simulink model "Simulink_DB2"  (R2012b)
settings: Solver=ode3  StartTime=0.0  StopTime=inf  FixedStep=0.001  RelTol=1e-3
undefined symbols (not defined in the file or in its folder): NULL
libraries: instrumentlib x3
settings Model: Creator=Petito  LastModifiedBy=Augusto
settings DataIOCC: SignalLoggingSaveFormat=ModelDataLogs
settings OptimizationCC: ExpressionDepthLimit=128
settings DebuggingCC: MultiTaskDSMMsg=warning  MultiTaskCondExecSysMsg=none  StrictBusMsg=None
settings HardwareCC: ProdIntDivRoundTo=Zero  ProdEndianess=LittleEndian  ProdHWDeviceType=Generic->32-bit x86 compatible
settings RTWCC: SystemTargetFile=rtwin.tlc  TemplateMakefile=rtwin.tmf  Description=Real-Time Windows Target  ProcessScript=rtwin_make_rtw_hook  IncludeERTFirstTime=on  RTWCompilerOptimization=On
settings CodeAppCC: MaxIdLength=95  CustomSymbolStrType=$N$R$M_T  InternalIdentifier=Shortened
settings TargetCC: TargetLibSuffix=_rtwin.lib  TargetPreCompLibLocation=C:\Program Files\MATLAB\R2013a\toolbox\rtw\targets\rtwin\lib\win64  CodeReplacementLibrary=ANSI_C  IsPILTarget=off  EnableShiftOperators=on

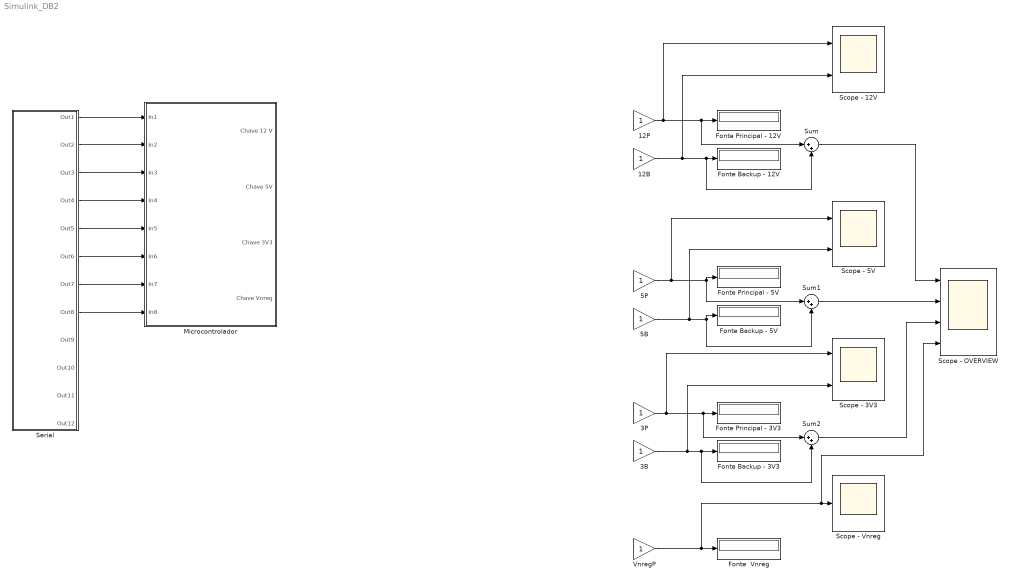
== system Simulink_DB2 ==
  12B : Gain
  12P : Gain
  3B : Gain
  3P : Gain
  5B : Gain
  5P : Gain
  Fonte  Vnreg : Display  mask(a){}
  Fonte Backup - 12V : Display
  Fonte Backup - 3V3 : Display
  Fonte Backup - 5V : Display
  Fonte Principal - 12V : Display  mask(a){}
  Fonte Principal - 3V3 : Display  mask(a){}
  Fonte Principal - 5V : Display  mask(a){}
  Microcontrolador : Subsystem
  Scope - 12V : Scope  NumInputPorts=2
      settings: TickLabels=on  TimeRange=10  YMin=0~0  YMax=13~13
  Scope - 3V3 : Scope  NumInputPorts=2
      settings: TickLabels=on  TimeRange=10  YMin=0~0  YMax=13~13  SaveName=ScopeData3
  Scope - 5V : Scope  NumInputPorts=2
      settings: TickLabels=on  TimeRange=10  YMin=0~0  YMax=6~6.5  SaveName=ScopeData2
  Scope - OVERVIEW : Scope  NumInputPorts=4
      settings: TickLabels=on  TimeRange=10  YMin=0~0~0~0  YMax=13~6~4~9
  Scope - Vnreg : Scope
      settings: TickLabels=on  TimeRange=10  YMin=0  YMax=13  SaveName=ScopeData4
  Serial : Subsystem
  Sum : Sum  Inputs=|++
  Sum1 : Sum  Inputs=|++
  Sum2 : Sum  Inputs=|++
  VnregP : Gain
  wires:
  ? -> VnregP/1
  ? -> 3P/1
  ? -> 3B/1
  ? -> 5P/1
  ? -> 5B/1
  ? -> 12B/1
  ? -> 12P/1
  12P/1 -> Scope - 12V/1, Fonte Principal - 12V/1, Sum/1
  12B/1 -> Scope - 12V/2, Sum/2, Fonte Backup - 12V/1
  5P/1 -> Scope - 5V/1, Fonte Principal - 5V/1, Sum1/1
  5B/1 -> Scope - 5V/2, Fonte Backup - 5V/1, Sum1/2
  VnregP/1 -> Scope - OVERVIEW/4, Scope - Vnreg/1, Fonte  Vnreg/1
  Serial/1(Out1) -> Microcontrolador/1(In1)
  Serial/2(Out2) -> Microcontrolador/2(In2)
  Serial/3(Out3) -> Microcontrolador/3(In3)
  Serial/4(Out4) -> Microcontrolador/4(In4)
  Serial/5(Out5) -> Microcontrolador/5(In5)
  Serial/6(Out6) -> Microcontrolador/6(In6)
  Serial/7(Out7) -> Microcontrolador/7(In7)
  Serial/8(Out8) -> Microcontrolador/8(In8)
  Sum/1 -> Scope - OVERVIEW/1
  Sum1/1 -> Scope - OVERVIEW/2
  3P/1 -> Scope - 3V3/1, Sum2/1, Fonte Principal - 3V3/1
  3B/1 -> Scope - 3V3/2, Sum2/2, Fonte Backup - 3V3/1
  Sum2/1 -> Scope - OVERVIEW/3

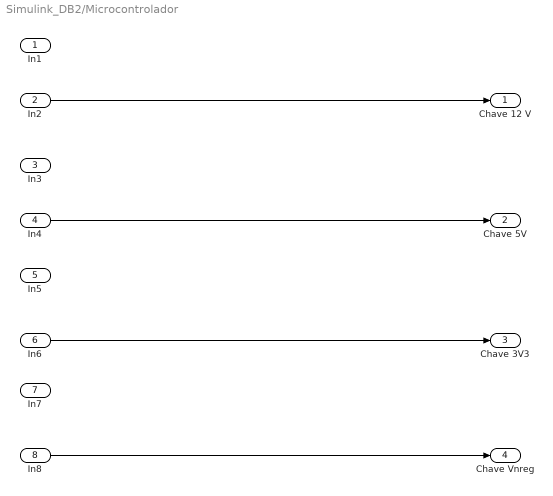
== system Simulink_DB2/Microcontrolador ==
  In1 : Inport
  In2 : Inport  Port=2
  In3 : Inport  Port=3
  In4 : Inport  Port=4
  In5 : Inport  Port=5
  In6 : Inport  Port=6
  In7 : Inport  Port=7
  In8 : Inport  Port=8
  Chave 12 V : Outport
  Chave 5V : Outport  Port=2
  Chave 3V3 : Outport  Port=3
  Chave Vnreg : Outport  Port=4
  wires:
  In4/1 -> Chave 5V/1
  In6/1 -> Chave 3V3/1
  In8/1 -> Chave Vnreg/1
  In2/1 -> Chave 12 V/1

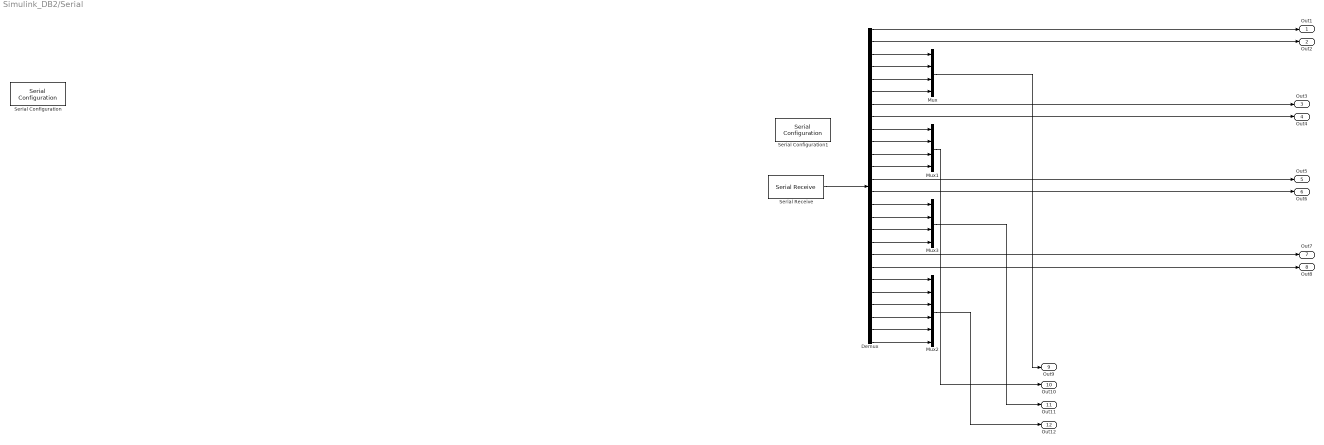
== system Simulink_DB2/Serial ==
  Demux : Demux  Outputs=26
  Mux : Mux
  Mux1 : Mux
  Mux2 : Mux  Inputs=6
  Mux3 : Mux
  Serial Configuration : instrumentlib/Serial Configuration  Priority=-200000  ComPortMenu=<Please select a port...>  ComPort=<Please select a port...>  BaudRate=115200  DataBits=8  Parity=none  StopBits=1  FlowControl=none  Timeout=10  ByteOrder=LittleEndian
  Serial Configuration1 : instrumentlib/Serial Configuration  Priority=-200000  ComPortMenu=<Please select a port...>  ComPort=<Please select a port...>  BaudRate=9600  DataBits=8  Parity=none  StopBits=1  FlowControl=none  Timeout=10  ByteOrder=LittleEndian
  Serial Receive : instrumentlib/Serial Receive  ComPortMenu=<Please select a port...>  ComPort=<Please select a port...>  Terminator=NULL ('\0')  DataSize="[1  26]"  DataType=int8  EnableBlockingMode=on  ActionDataUnavailable=Output last received value  CustomValue=0  SampleTime=0.01
  Out1 : Outport
  Out2 : Outport  Port=2
  Out3 : Outport  Port=3
  Out4 : Outport  Port=4
  Out5 : Outport  Port=5
  Out6 : Outport  Port=6
  Out7 : Outport  Port=7
  Out8 : Outport  Port=8
  Out9 : Outport  Port=9
  Out10 : Outport  Port=10
  Out11 : Outport  Port=11
  Out12 : Outport  Port=12
  wires:
  Mux3/1 -> Out11/1
  Demux/21 -> Mux2/1
  Demux/22 -> Mux2/2
  Demux/25 -> Mux2/5
  Demux/20 -> Out8/1
  Demux/13 -> Out5/1
  Mux1/1 -> Out10/1
  Mux/1 -> Out9/1
  Serial Receive/1 -> Demux/1
  Demux/26 -> Mux2/6
  Demux/24 -> Mux2/4
  Demux/23 -> Mux2/3
  Demux/10 -> Mux1/2
  Demux/17 -> Mux3/3
  Demux/18 -> Mux3/4
  Demux/12 -> Mux1/4
  Demux/5 -> Mux/3
  Demux/16 -> Mux3/2
  Demux/15 -> Mux3/1
  Demux/6 -> Mux/4
  Demux/9 -> Mux1/1
  Demux/4 -> Mux/2
  Demux/3 -> Mux/1
  Demux/11 -> Mux1/3
  Demux/2 -> Out2/1
  Demux/1 -> Out1/1
  Demux/8 -> Out4/1
  Demux/14 -> Out6/1
  Demux/19 -> Out7/1
  Demux/7 -> Out3/1
  Mux2/1 -> Out12/1
